simulink model "sensorExpolerEncoder"  (R2026a)
settings: Solver=FixedStepDiscrete  StopTime=inf  FixedStep=0.001
undefined symbols (not defined in the file): Blocking, Non
libraries: amg_usbconverter_n_connect_lib x2, simulink x1
settings Model: Creator=pboon  LastModifiedBy=focus

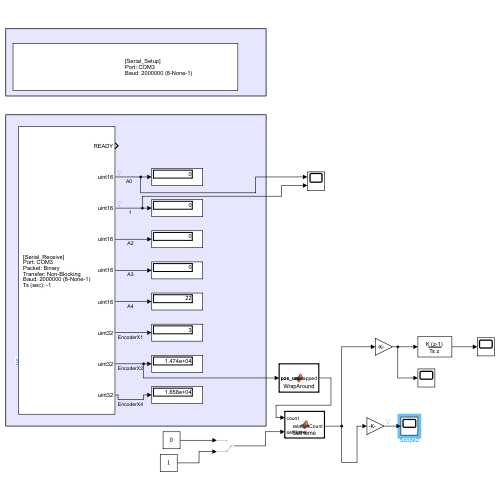
[thumbnail: Simulink's stored preview of the top-level diagram]
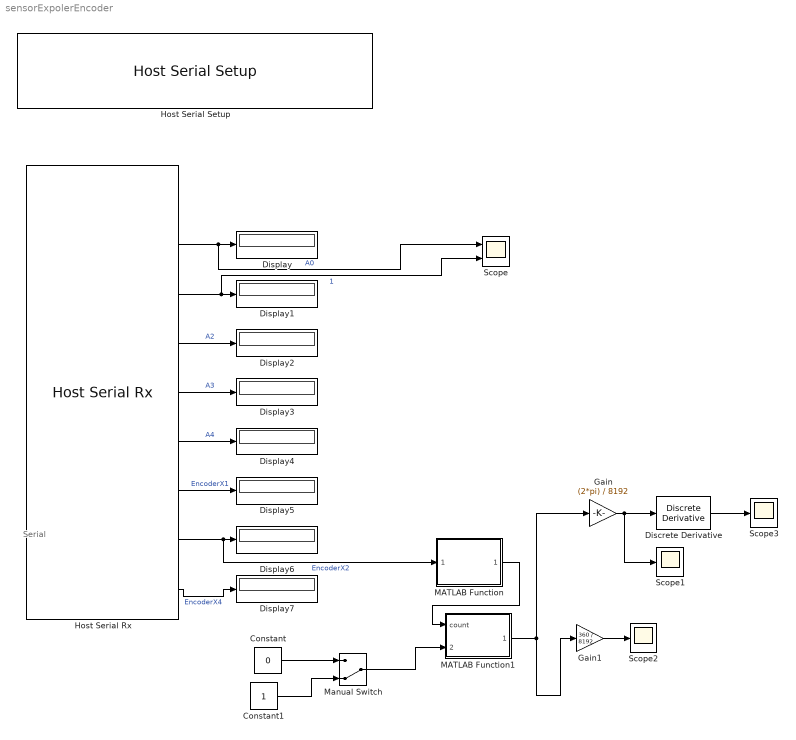
== system sensorExpolerEncoder ==
  note: Serial
  Constant : Constant  Value=0
  Constant1 : Constant
  Discrete Derivative : simulink/Discrete/Discrete Derivative  gainval=1.0  ICPrevScaledInput=0.0  OutMin=[]  OutMax=[]  OutDataType=fixdt(1, 16)  OutScaling=2^-10  DoSatur=off
  Display{,1..7} (8 alike) : Display
  Gain : Gain  Gain=(2*pi) / 8192
  Gain1 : Gain  Gain=360 / 8192
  Host Serial Rx : amg_usbconverter_n_connect_lib/Host Serial Rx  conf=rx  port=COM3  baudrate=2000000  databits=8  parity=None  stopbit=1  flowcontrol=None  transfer=Non-Blocking  timeout=5  packetmode=Binary  enableinitialvalues=off  initialvalues=[]  binheader='25'  binterminator='4E 4E'  porttype_double=0  porttype_single=0  porttype_int8=0  porttype_uint8=0  porttype_int16=0  porttype_uint16=5  porttype_int32=0  porttype_uint32=3  asciiformat='%d,%f'  rx_asciiterminator="CRLF (0x0D 0x0A - \"\\r\\n\")"  tx_asciiterminator="CRLF (0x0D 0x0A - \"\\r\\n\")"  sampletime=0.001  enablecustomportlabel=off  cinputportlabel=0  coutputportlabel=A  portpinstr=0  blockid=HostSerialRx  inputporttype=[]  inputportwidth=[]  inputportlabel={}  outputporttype=[3 5 5 5 5 5 7 7 7]  outputportwidth=[1 1 1 1 1 1 1 1 1]  outputportlabel={'READY','uint16','uint16','uint16','uint16','uint16','uint32','uint32','uint32'}  compat=0  optionstring=[]  autoport='COM3'
  Host Serial Setup : amg_usbconverter_n_connect_lib/Host Serial Setup  conf=setup  port=COM3  baudrate=2000000  databits=8  parity=None  stopbit=1  flowcontrol=None  transfer=Blocking  timeout=2  packetmode=Binary  initialvalues=[]  binheader='7E 7E'  binterminator='03 03'  porttype_double=0  porttype_single=1  porttype_int8=0  porttype_uint8=0  porttype_int16=0  porttype_uint16=0  porttype_int32=0  porttype_uint32=2  asciiformat='%d %u %x'  rx_asciiterminator="CRLF (0x0D 0x0A - \"\\r\\n\")"  tx_asciiterminator="CRLF (0x0D 0x0A - \"\\r\\n\")"  sampletime=-1  enablecustomportlabel=off  cinputportlabel=0  coutputportlabel=A  portpinstr=0  blockid=HostSerialSetup  inputporttype=[]  inputportwidth=[]  inputportlabel={}  outputporttype=[]  outputportwidth=[]  outputportlabel={}  compat=0  optionstring=[]  autoport='COM3'
  MATLAB Function : MATLAB Function  TreatAsAtomicUnit=on
  MATLAB Function1 : MATLAB Function  TreatAsAtomicUnit=on
  Manual Switch : ManualSwitch  CurrentSetting=0
  Scope : Scope  NumInputPorts=2
      settings: ActiveDisplayYMinimum=-3607.5475855121649  ActiveDisplayYMaximum=7033.9660328497748
  Scope1 : Scope
  Scope2 : Scope
      settings: ActiveDisplayYMinimum=-1282.2868556376095  ActiveDisplayYMaximum=1595.9329598282895  DataLoggingVariableName=ScopeData2
  Scope3 : Scope
      settings: ActiveDisplayYMinimum=-1  ActiveDisplayYMaximum=1  DataLoggingVariableName=ScopeData3
  wires:
  Host Serial Rx/2 -> Scope/1, Display/1  "A0"
  Host Serial Rx/3 -> Scope/2, Display1/1  "1"
  Host Serial Rx/4 -> Display2/1  "A2"
  Host Serial Rx/5 -> Display3/1  "A3"
  Host Serial Rx/6 -> Display4/1  "A4"
  Host Serial Rx/7 -> Display5/1  "EncoderX1"
  Host Serial Rx/8 -> MATLAB Function/1(pos_raw), Display6/1  "EncoderX2"
  Host Serial Rx/9 -> Display7/1  "EncoderX4"
  MATLAB Function/1(pos_unwrapped) -> MATLAB Function1/1(count)
  Gain/1 -> Scope1/1, Discrete Derivative/1
  Gain1/1 -> Scope2/1
  Discrete Derivative/1 -> Scope3/1
  MATLAB Function1/1(relativeCount) -> Gain1/1, Gain/1
  Constant/1 -> Manual Switch/1
  Constant1/1 -> Manual Switch/2
  Manual Switch/1 -> MATLAB Function1/2(setHome)

== matlab function sensorExpolerEncoder/MATLAB Function ==
  data: pos_raw input; pos_unwrapped output
function pos_unwrapped = WrapAround(pos_raw)
    % แปลงค่า pos_raw เป็น double ทันทีเพื่อป้องกันปัญหา uint32 ลบแล้วติดลบไม่ได้
    pos_curr = double(pos_raw);
    
    persistent pos_prev offset
    
    if isempty(pos_prev)
        pos_prev = pos_curr;
        offset = 0;
    end
    
    % ตั้งค่า Counter Period ตามโจทย์แล็บ (0 ถึง 61439)
    MAX_PERIOD = 61439;
    
    diff = pos_curr - pos_prev;
    
    % ตรวจสอบการเกิด Overflow
    if diff < -MAX_PERIOD / 2
        offset = offset + (MAX_PERIOD + 1); % เพิ่ม offset ชดเชยเท่ากับ 61440
    elseif diff > MAX_PERIOD / 2
        offset = offset - (MAX_PERIOD + 1);
    end
    
    pos_unwrapped = pos_curr + offset;
    pos_prev = pos_curr;
end

== matlab function sensorExpolerEncoder/MATLAB Function1 ==
  data: count input; relativeCount output; setHome input
function relativeCount = SetHome(count, setHome)
%#codegen

persistent homeOffset prevSetHome

if isempty(homeOffset)
    homeOffset = double(0);
end

if isempty(prevSetHome)
    prevSetHome = double(0);
end

% Detect rising edge: 0 -> 1
if (setHome == 1) && (prevSetHome == 0)
    homeOffset = double(count);
end

relativeCount = double(count) - homeOffset;

prevSetHome = setHome;
end
